simulink model "project"  (R2018b)
settings: Solver=VariableStepAuto  StartTime=0.0  StopTime=10.0  RelTol=1e-3
libraries: commutil2 x4
(part 1 of 2)
settings Model: Creator=Reza  LastModifiedBy=Rahmat

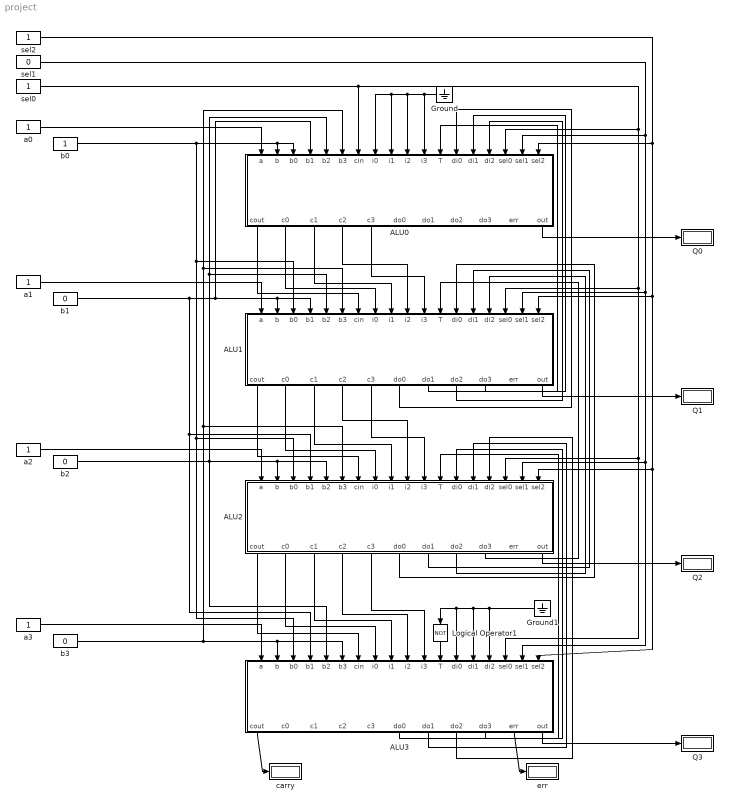
== system project ==
  ALU0 : Subsystem
  ALU1 : Subsystem
  ALU2 : Subsystem
  ALU3 : Subsystem
  Ground : Ground
  Ground1 : Ground
  Logical Operator1 : Logic  Operator=NOT  IconShape=distinctive  AllPortsSameDT=off  OutDataTypeStr=boolean
  Q{0..3} (4 alike) : Display
  a{0..3} (4 alike) : Constant
  b0 : Constant
  b1 : Constant  Value=0
  b2 : Constant  Value=0
  b3 : Constant  Value=0
  carry : Display
  err : Display
  sel0 : Constant
  sel1 : Constant  Value=0
  sel2 : Constant
  wires:
  ALU0/11(out) -> Q0/1
  sel0/1 -> ALU0/7(cin), ALU0/16(sel0), ALU1/16(sel0), ALU2/16(sel0), ALU3/16(sel0)
  sel1/1 -> ALU0/17(sel1), ALU1/17(sel1), ALU2/17(sel1), ALU3/17(sel1)
  sel2/1 -> ALU0/18(sel2), ALU1/18(sel2), ALU2/18(sel2), ALU3/18(sel2)
  ALU1/11(out) -> Q1/1
  ALU2/11(out) -> Q2/1
  ALU3/11(out) -> Q3/1
  a0/1 -> ALU0/1(a)
  a1/1 -> ALU1/1(a)
  a2/1 -> ALU2/1(a)
  a3/1 -> ALU3/1(a)
  b0/1 -> ALU3/3(b0), ALU2/3(b0), ALU1/3(b0), ALU0/3(b0), ALU0/2(b)
  b2/1 -> ALU2/5(b2), ALU2/2(b), ALU3/5(b2), ALU0/5(b2), ALU1/5(b2)
  b3/1 -> ALU3/6(b3), ALU3/2(b), ALU2/6(b3), ALU0/6(b3), ALU1/6(b3)
  b1/1 -> ALU1/4(b1), ALU1/2(b), ALU0/4(b1), ALU3/4(b1), ALU2/4(b1)
  ALU0/1(cout) -> ALU1/7(cin)
  ALU1/1(cout) -> ALU2/7(cin)
  ALU2/1(cout) -> ALU3/7(cin)
  ALU3/1(cout) -> carry/1
  ALU3/10(err) -> err/1
  ALU0/2(c0) -> ALU1/8(i0)
  ALU0/3(c1) -> ALU1/9(i1)
  ALU0/4(c2) -> ALU1/10(i2)
  ALU0/5(c3) -> ALU1/11(i3)
  ALU1/2(c0) -> ALU2/8(i0)
  ALU1/3(c1) -> ALU2/9(i1)
  ALU1/4(c2) -> ALU2/10(i2)
  ALU1/5(c3) -> ALU2/11(i3)
  ALU2/2(c0) -> ALU3/8(i0)
  ALU2/3(c1) -> ALU3/9(i1)
  ALU2/4(c2) -> ALU3/10(i2)
  ALU2/5(c3) -> ALU3/11(i3)
  Ground/1 -> ALU0/11(i3), ALU0/10(i2), ALU0/9(i1), ALU0/8(i0)
  Ground1/1 -> ALU3/14(di1), ALU3/13(di0), Logical Operator1/1, ALU3/15(di2)
  Logical Operator1/1 -> ALU3/12(T)
  ALU3/9(do3) -> ALU2/12(T)
  ALU3/6(do0) -> ALU2/13(di0)
  ALU3/7(do1) -> ALU2/14(di1)
  ALU3/8(do2) -> ALU2/15(di2)
  ALU2/9(do3) -> ALU1/12(T)
  ALU2/8(do2) -> ALU1/15(di2)
  ALU2/7(do1) -> ALU1/14(di1)
  ALU2/6(do0) -> ALU1/13(di0)
  ALU1/9(do3) -> ALU0/12(T)
  ALU1/8(do2) -> ALU0/15(di2)
  ALU1/7(do1) -> ALU0/14(di1)
  ALU1/6(do0) -> ALU0/13(di0)

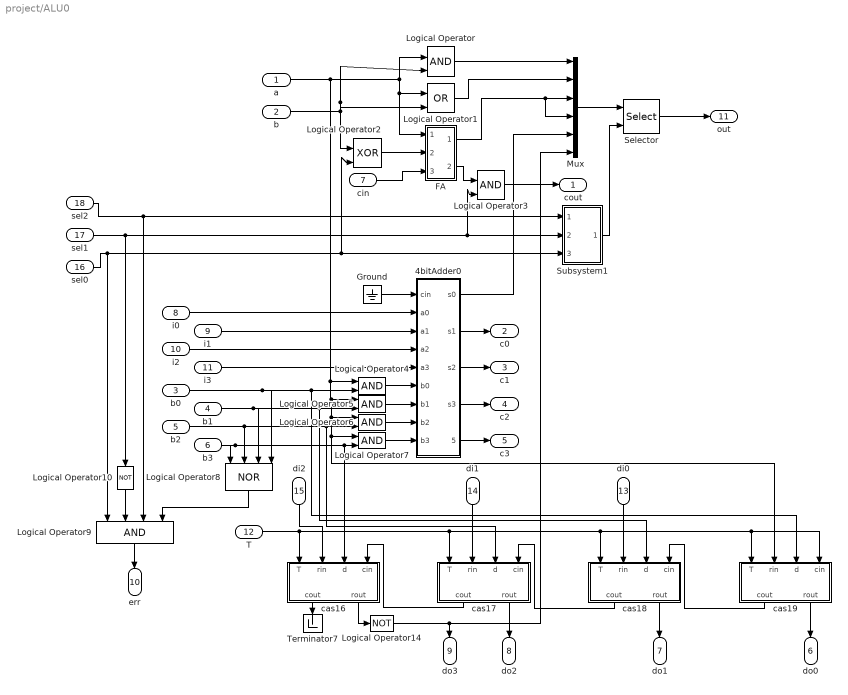
== system project/ALU0 ==
  a : Inport
  b : Inport  Port=2
  b0 : Inport  Port=3
  b1 : Inport  Port=4
  b2 : Inport  Port=5
  b3 : Inport  Port=6
  cin : Inport  Port=7
  i0 : Inport  Port=8
  i1 : Inport  Port=9
  i2 : Inport  Port=10
  i3 : Inport  Port=11
  T : Inport  Port=12
  di0 : Inport  Port=13
  di1 : Inport  Port=14
  di2 : Inport  Port=15
  sel0 : Inport  Port=16
  sel1 : Inport  Port=17
  sel2 : Inport  Port=18
  4bitAdder0 : Subsystem
  FA : Subsystem
  Ground : Ground
  Logical Operator{,3..7} (6 alike) : Logic  IconShape=distinctive  AllPortsSameDT=off  OutDataTypeStr=boolean
  Logical Operator1 : Logic  Operator=OR  IconShape=distinctive  AllPortsSameDT=off  OutDataTypeStr=boolean
  Logical Operator10 : Logic  Operator=NOT  IconShape=distinctive  AllPortsSameDT=off  OutDataTypeStr=boolean
  Logical Operator14 : Logic  Operator=NOT  IconShape=distinctive  AllPortsSameDT=off  OutDataTypeStr=boolean
  Logical Operator2 : Logic  Operator=XOR  IconShape=distinctive  AllPortsSameDT=off  OutDataTypeStr=boolean
  Logical Operator8 : Logic  Operator=NOR  Inputs=4  IconShape=distinctive  AllPortsSameDT=off  OutDataTypeStr=boolean
  Logical Operator9 : Logic  Inputs=4  IconShape=distinctive  AllPortsSameDT=off  OutDataTypeStr=boolean
  Mux : Mux  Inputs=6
  Selector : Selector  InputPortWidth=6  IndexOptions=Starting index (port)  Indices=[1 3]  OutputSizes=1
  Subsystem1 : Subsystem
  Terminator7 : Terminator
  cas16 : Subsystem
  cas17 : Subsystem
  cas18 : Subsystem
  cas19 : Subsystem
  cout : Outport
  c0 : Outport  Port=2
  c1 : Outport  Port=3
  c2 : Outport  Port=4
  c3 : Outport  Port=5
  do0 : Outport  Port=6
  do1 : Outport  Port=7
  do2 : Outport  Port=8
  do3 : Outport  Port=9
  err : Outport  Port=10
  out : Outport  Port=11
  wires:
  b/1 -> Logical Operator/2, Logical Operator1/2, Logical Operator2/1
  Mux/1 -> Selector/1
  sel1/1 -> Logical Operator10/1, Logical Operator3/2, Subsystem1/2(sel1)
  FA/1(Out2) -> Mux/3, Mux/4
  sel2/1 -> Logical Operator9/3, Subsystem1/1(sel2)
  Subsystem1/1(Out1) -> Selector/2
  a/1 -> Logical Operator7/1, cas19/2(rin), Logical Operator6/1, Logical Operator5/1, Logical Operator4/1, FA/1(In2), Logical Operator1/1, Logical Operator/1
  cin/1 -> FA/3(In4)
  Logical Operator2/1 -> FA/2(In3)
  Selector/1 -> out/1
  sel0/1 -> Logical Operator9/1, Logical Operator2/2, Subsystem1/3(sel0)
  Logical Operator1/1 -> Mux/2
  Logical Operator/1 -> Mux/1
  FA/2(Out1) -> Logical Operator3/1
  Logical Operator3/1 -> cout/1
  4bitAdder0/1(s0) -> Mux/5
  i0/1 -> 4bitAdder0/2(a0)
  i1/1 -> 4bitAdder0/3(a1)
  i2/1 -> 4bitAdder0/4(a2)
  i3/1 -> 4bitAdder0/5(a3)
  Logical Operator4/1 -> 4bitAdder0/6(b0)
  Logical Operator5/1 -> 4bitAdder0/7(b1)
  4bitAdder0/2(s1) -> c0/1
  4bitAdder0/3(s2) -> c1/1
  4bitAdder0/4(s3) -> c2/1
  4bitAdder0/5(cout) -> c3/1
  Logical Operator6/1 -> 4bitAdder0/8(b2)
  Logical Operator7/1 -> 4bitAdder0/9(b3)
  b0/1 -> Logical Operator8/4, Logical Operator4/2, cas19/3(d)
  b1/1 -> Logical Operator8/3, Logical Operator5/2, cas18/3(d)
  b2/1 -> Logical Operator8/2, cas17/3(d), Logical Operator6/2
  b3/1 -> Logical Operator8/1, cas16/3(d), Logical Operator7/2
  cas19/1(cout) -> cas18/4(cin)
  cas18/1(cout) -> cas17/4(cin)
  cas17/1(cout) -> cas16/4(cin)
  cas16/1(cout) -> Terminator7/1
  T/1 -> cas16/1(T), cas17/1(T), cas18/1(T), cas19/1(T), cas19/4(cin)
  cas16/2(rout) -> Logical Operator14/1
  Logical Operator14/1 -> do3/1, Mux/6
  di0/1 -> cas18/2(rin)
  di1/1 -> cas17/2(rin)
  di2/1 -> cas16/2(rin)
  cas19/2(rout) -> do0/1
  cas18/2(rout) -> do1/1
  cas17/2(rout) -> do2/1
  Ground/1 -> 4bitAdder0/1(cin)
  Logical Operator9/1 -> err/1
  Logical Operator8/1 -> Logical Operator9/4
  Logical Operator10/1 -> Logical Operator9/2

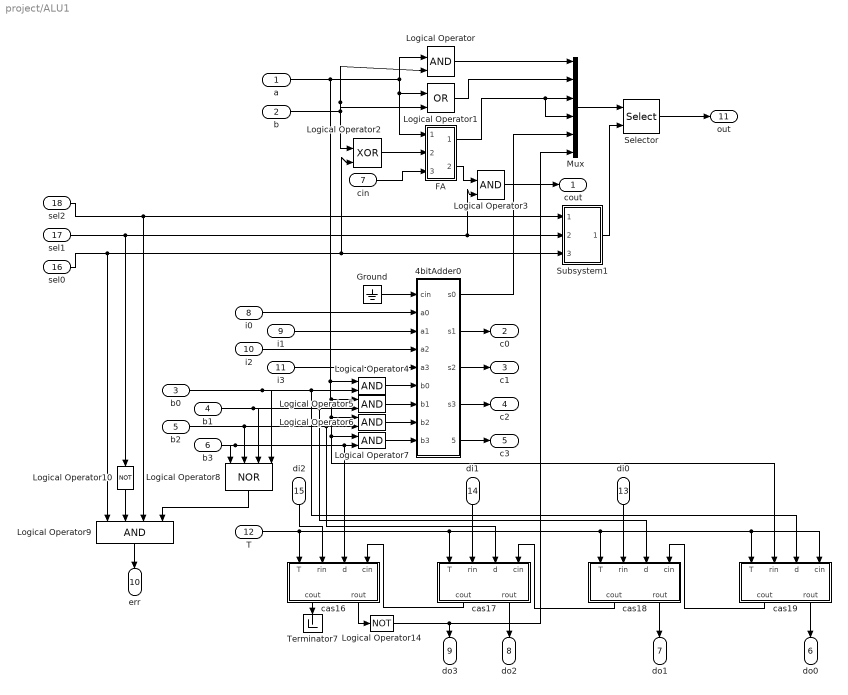
== system project/ALU1 ==
  a : Inport
  b : Inport  Port=2
  b0 : Inport  Port=3
  b1 : Inport  Port=4
  b2 : Inport  Port=5
  b3 : Inport  Port=6
  cin : Inport  Port=7
  i0 : Inport  Port=8
  i1 : Inport  Port=9
  i2 : Inport  Port=10
  i3 : Inport  Port=11
  T : Inport  Port=12
  di0 : Inport  Port=13
  di1 : Inport  Port=14
  di2 : Inport  Port=15
  sel0 : Inport  Port=16
  sel1 : Inport  Port=17
  sel2 : Inport  Port=18
  4bitAdder0 : Subsystem
  FA : Subsystem
  Ground : Ground
  Logical Operator{,3..7} (6 alike) : Logic  IconShape=distinctive  AllPortsSameDT=off  OutDataTypeStr=boolean
  Logical Operator1 : Logic  Operator=OR  IconShape=distinctive  AllPortsSameDT=off  OutDataTypeStr=boolean
  Logical Operator10 : Logic  Operator=NOT  IconShape=distinctive  AllPortsSameDT=off  OutDataTypeStr=boolean
  Logical Operator14 : Logic  Operator=NOT  IconShape=distinctive  AllPortsSameDT=off  OutDataTypeStr=boolean
  Logical Operator2 : Logic  Operator=XOR  IconShape=distinctive  AllPortsSameDT=off  OutDataTypeStr=boolean
  Logical Operator8 : Logic  Operator=NOR  Inputs=4  IconShape=distinctive  AllPortsSameDT=off  OutDataTypeStr=boolean
  Logical Operator9 : Logic  Inputs=4  IconShape=distinctive  AllPortsSameDT=off  OutDataTypeStr=boolean
  Mux : Mux  Inputs=6
  Selector : Selector  InputPortWidth=6  IndexOptions=Starting index (port)  Indices=[1 3]  OutputSizes=1
  Subsystem1 : Subsystem
  Terminator7 : Terminator
  cas16 : Subsystem
  cas17 : Subsystem
  cas18 : Subsystem
  cas19 : Subsystem
  cout : Outport
  c0 : Outport  Port=2
  c1 : Outport  Port=3
  c2 : Outport  Port=4
  c3 : Outport  Port=5
  do0 : Outport  Port=6
  do1 : Outport  Port=7
  do2 : Outport  Port=8
  do3 : Outport  Port=9
  err : Outport  Port=10
  out : Outport  Port=11
  wires:
  b/1 -> Logical Operator/2, Logical Operator1/2, Logical Operator2/1
  Mux/1 -> Selector/1
  FA/1(Out2) -> Mux/3, Mux/4
  Subsystem1/1(Out1) -> Selector/2
  a/1 -> Logical Operator7/1, cas19/2(rin), Logical Operator6/1, Logical Operator5/1, Logical Operator4/1, FA/1(In2), Logical Operator1/1, Logical Operator/1
  cin/1 -> FA/3(In4)
  Logical Operator2/1 -> FA/2(In3)
  Selector/1 -> out/1
  Logical Operator1/1 -> Mux/2
  Logical Operator/1 -> Mux/1
  FA/2(Out1) -> Logical Operator3/1
  Logical Operator3/1 -> cout/1
  4bitAdder0/1(s0) -> Mux/5
  i0/1 -> 4bitAdder0/2(a0)
  i1/1 -> 4bitAdder0/3(a1)
  i2/1 -> 4bitAdder0/4(a2)
  i3/1 -> 4bitAdder0/5(a3)
  Logical Operator4/1 -> 4bitAdder0/6(b0)
  Logical Operator5/1 -> 4bitAdder0/7(b1)
  4bitAdder0/2(s1) -> c0/1
  4bitAdder0/3(s2) -> c1/1
  4bitAdder0/4(s3) -> c2/1
  4bitAdder0/5(cout) -> c3/1
  Logical Operator6/1 -> 4bitAdder0/8(b2)
  Logical Operator7/1 -> 4bitAdder0/9(b3)
  b0/1 -> Logical Operator8/4, Logical Operator4/2, cas19/3(d)
  b1/1 -> Logical Operator8/3, Logical Operator5/2, cas18/3(d)
  b2/1 -> Logical Operator8/2, cas17/3(d), Logical Operator6/2
  b3/1 -> Logical Operator8/1, cas16/3(d), Logical Operator7/2
  cas19/1(cout) -> cas18/4(cin)
  cas18/1(cout) -> cas17/4(cin)
  cas17/1(cout) -> cas16/4(cin)
  cas16/1(cout) -> Terminator7/1
  T/1 -> cas16/1(T), cas17/1(T), cas18/1(T), cas19/1(T), cas19/4(cin)
  cas16/2(rout) -> Logical Operator14/1
  Logical Operator14/1 -> do3/1, Mux/6
  di0/1 -> cas18/2(rin)
  di1/1 -> cas17/2(rin)
  di2/1 -> cas16/2(rin)
  cas19/2(rout) -> do0/1
  cas18/2(rout) -> do1/1
  cas17/2(rout) -> do2/1
  Ground/1 -> 4bitAdder0/1(cin)
  sel2/1 -> Logical Operator9/3, Subsystem1/1(sel2)
  sel0/1 -> Logical Operator9/1, Logical Operator2/2, Subsystem1/3(sel0)
  Logical Operator10/1 -> Logical Operator9/2
  Logical Operator9/1 -> err/1
  Logical Operator8/1 -> Logical Operator9/4
  sel1/1 -> Logical Operator10/1, Logical Operator3/2, Subsystem1/2(sel1)

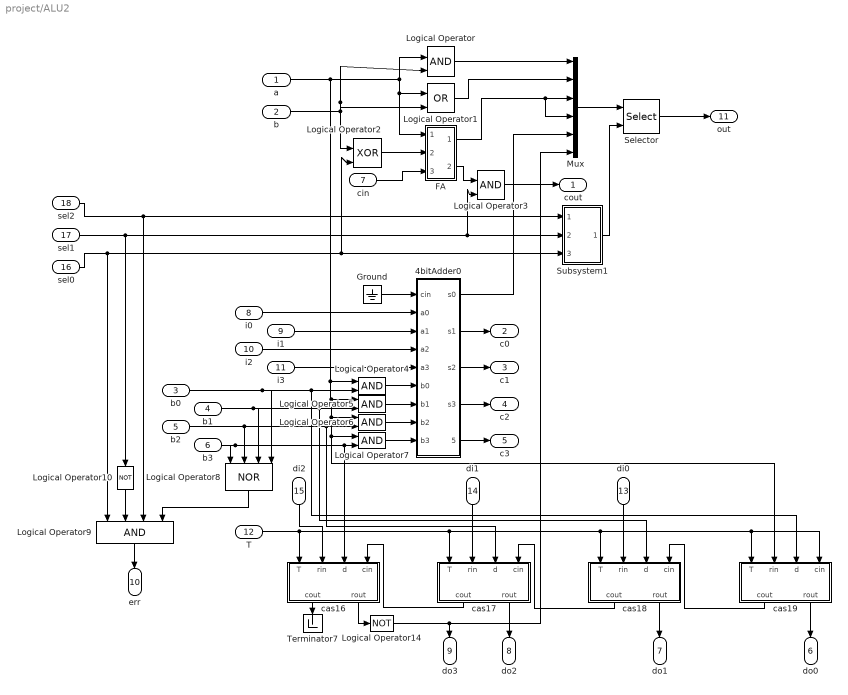
== system project/ALU2 ==
  a : Inport
  b : Inport  Port=2
  b0 : Inport  Port=3
  b1 : Inport  Port=4
  b2 : Inport  Port=5
  b3 : Inport  Port=6
  cin : Inport  Port=7
  i0 : Inport  Port=8
  i1 : Inport  Port=9
  i2 : Inport  Port=10
  i3 : Inport  Port=11
  T : Inport  Port=12
  di0 : Inport  Port=13
  di1 : Inport  Port=14
  di2 : Inport  Port=15
  sel0 : Inport  Port=16
  sel1 : Inport  Port=17
  sel2 : Inport  Port=18
  4bitAdder0 : Subsystem
  FA : Subsystem
  Ground : Ground
  Logical Operator{,3..7} (6 alike) : Logic  IconShape=distinctive  AllPortsSameDT=off  OutDataTypeStr=boolean
  Logical Operator1 : Logic  Operator=OR  IconShape=distinctive  AllPortsSameDT=off  OutDataTypeStr=boolean
  Logical Operator10 : Logic  Operator=NOT  IconShape=distinctive  AllPortsSameDT=off  OutDataTypeStr=boolean
  Logical Operator14 : Logic  Operator=NOT  IconShape=distinctive  AllPortsSameDT=off  OutDataTypeStr=boolean
  Logical Operator2 : Logic  Operator=XOR  IconShape=distinctive  AllPortsSameDT=off  OutDataTypeStr=boolean
  Logical Operator8 : Logic  Operator=NOR  Inputs=4  IconShape=distinctive  AllPortsSameDT=off  OutDataTypeStr=boolean
  Logical Operator9 : Logic  Inputs=4  IconShape=distinctive  AllPortsSameDT=off  OutDataTypeStr=boolean
  Mux : Mux  Inputs=6
  Selector : Selector  InputPortWidth=6  IndexOptions=Starting index (port)  Indices=[1 3]  OutputSizes=1
  Subsystem1 : Subsystem
  Terminator7 : Terminator
  cas16 : Subsystem
  cas17 : Subsystem
  cas18 : Subsystem
  cas19 : Subsystem
  cout : Outport
  c0 : Outport  Port=2
  c1 : Outport  Port=3
  c2 : Outport  Port=4
  c3 : Outport  Port=5
  do0 : Outport  Port=6
  do1 : Outport  Port=7
  do2 : Outport  Port=8
  do3 : Outport  Port=9
  err : Outport  Port=10
  out : Outport  Port=11
  wires:
  b/1 -> Logical Operator/2, Logical Operator1/2, Logical Operator2/1
  Mux/1 -> Selector/1
  FA/1(Out2) -> Mux/3, Mux/4
  Subsystem1/1(Out1) -> Selector/2
  a/1 -> Logical Operator7/1, cas19/2(rin), Logical Operator6/1, Logical Operator5/1, Logical Operator4/1, FA/1(In2), Logical Operator1/1, Logical Operator/1
  cin/1 -> FA/3(In4)
  Logical Operator2/1 -> FA/2(In3)
  Selector/1 -> out/1
  Logical Operator1/1 -> Mux/2
  Logical Operator/1 -> Mux/1
  FA/2(Out1) -> Logical Operator3/1
  Logical Operator3/1 -> cout/1
  4bitAdder0/1(s0) -> Mux/5
  i0/1 -> 4bitAdder0/2(a0)
  i1/1 -> 4bitAdder0/3(a1)
  i2/1 -> 4bitAdder0/4(a2)
  i3/1 -> 4bitAdder0/5(a3)
  Logical Operator4/1 -> 4bitAdder0/6(b0)
  Logical Operator5/1 -> 4bitAdder0/7(b1)
  4bitAdder0/2(s1) -> c0/1
  4bitAdder0/3(s2) -> c1/1
  4bitAdder0/4(s3) -> c2/1
  4bitAdder0/5(cout) -> c3/1
  Logical Operator6/1 -> 4bitAdder0/8(b2)
  Logical Operator7/1 -> 4bitAdder0/9(b3)
  b0/1 -> Logical Operator8/4, Logical Operator4/2, cas19/3(d)
  b1/1 -> Logical Operator8/3, Logical Operator5/2, cas18/3(d)
  b2/1 -> Logical Operator8/2, cas17/3(d), Logical Operator6/2
  b3/1 -> Logical Operator8/1, cas16/3(d), Logical Operator7/2
  cas19/1(cout) -> cas18/4(cin)
  cas18/1(cout) -> cas17/4(cin)
  cas17/1(cout) -> cas16/4(cin)
  cas16/1(cout) -> Terminator7/1
  T/1 -> cas16/1(T), cas17/1(T), cas18/1(T), cas19/1(T), cas19/4(cin)
  cas16/2(rout) -> Logical Operator14/1
  Logical Operator14/1 -> do3/1, Mux/6
  di0/1 -> cas18/2(rin)
  di1/1 -> cas17/2(rin)
  di2/1 -> cas16/2(rin)
  cas19/2(rout) -> do0/1
  cas18/2(rout) -> do1/1
  cas17/2(rout) -> do2/1
  Ground/1 -> 4bitAdder0/1(cin)
  sel2/1 -> Subsystem1/1(sel2), Logical Operator9/3
  sel0/1 -> Logical Operator9/1, Logical Operator2/2, Subsystem1/3(sel0)
  Logical Operator10/1 -> Logical Operator9/2
  Logical Operator9/1 -> err/1
  Logical Operator8/1 -> Logical Operator9/4
  sel1/1 -> Logical Operator3/2, Subsystem1/2(sel1), Logical Operator10/1

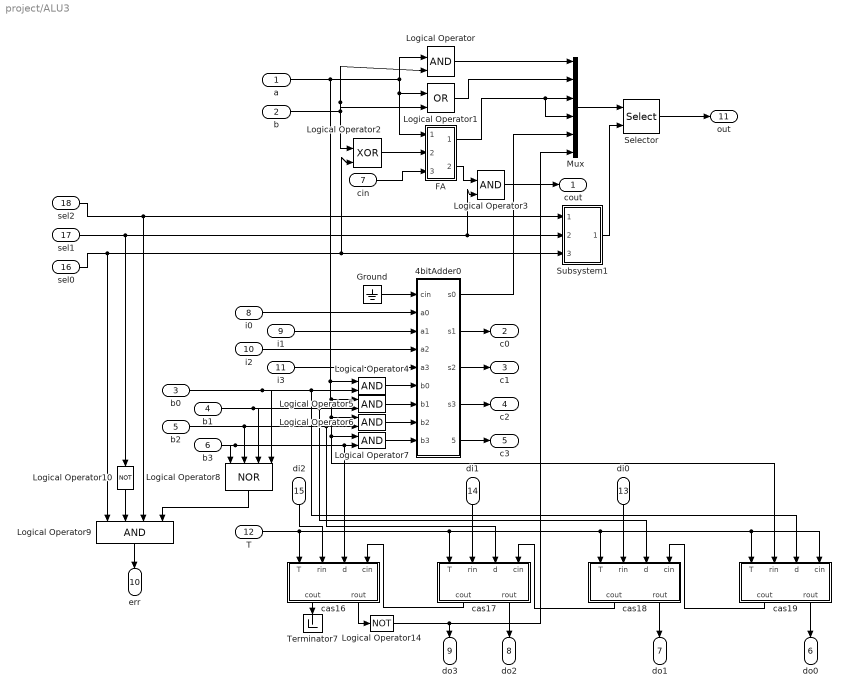
== system project/ALU3 ==
  a : Inport
  b : Inport  Port=2
  b0 : Inport  Port=3
  b1 : Inport  Port=4
  b2 : Inport  Port=5
  b3 : Inport  Port=6
  cin : Inport  Port=7
  i0 : Inport  Port=8
  i1 : Inport  Port=9
  i2 : Inport  Port=10
  i3 : Inport  Port=11
  T : Inport  Port=12
  di0 : Inport  Port=13
  di1 : Inport  Port=14
  di2 : Inport  Port=15
  sel0 : Inport  Port=16
  sel1 : Inport  Port=17
  sel2 : Inport  Port=18
  4bitAdder0 : Subsystem
  FA : Subsystem
  Ground : Ground
  Logical Operator{,3..7} (6 alike) : Logic  IconShape=distinctive  AllPortsSameDT=off  OutDataTypeStr=boolean
  Logical Operator1 : Logic  Operator=OR  IconShape=distinctive  AllPortsSameDT=off  OutDataTypeStr=boolean
  Logical Operator10 : Logic  Operator=NOT  IconShape=distinctive  AllPortsSameDT=off  OutDataTypeStr=boolean
  Logical Operator14 : Logic  Operator=NOT  IconShape=distinctive  AllPortsSameDT=off  OutDataTypeStr=boolean
  Logical Operator2 : Logic  Operator=XOR  IconShape=distinctive  AllPortsSameDT=off  OutDataTypeStr=boolean
  Logical Operator8 : Logic  Operator=NOR  Inputs=4  IconShape=distinctive  AllPortsSameDT=off  OutDataTypeStr=boolean
  Logical Operator9 : Logic  Inputs=4  IconShape=distinctive  AllPortsSameDT=off  OutDataTypeStr=boolean
  Mux : Mux  Inputs=6
  Selector : Selector  InputPortWidth=6  IndexOptions=Starting index (port)  Indices=[1 3]  OutputSizes=1
  Subsystem1 : Subsystem
  Terminator7 : Terminator
  cas16 : Subsystem
  cas17 : Subsystem
  cas18 : Subsystem
  cas19 : Subsystem
  cout : Outport
  c0 : Outport  Port=2
  c1 : Outport  Port=3
  c2 : Outport  Port=4
  c3 : Outport  Port=5
  do0 : Outport  Port=6
  do1 : Outport  Port=7
  do2 : Outport  Port=8
  do3 : Outport  Port=9
  err : Outport  Port=10
  out : Outport  Port=11
  wires:
  b/1 -> Logical Operator/2, Logical Operator1/2, Logical Operator2/1
  Mux/1 -> Selector/1
  FA/1(Out2) -> Mux/3, Mux/4
  Subsystem1/1(Out1) -> Selector/2
  a/1 -> Logical Operator7/1, cas19/2(rin), Logical Operator6/1, Logical Operator5/1, Logical Operator4/1, FA/1(In2), Logical Operator1/1, Logical Operator/1
  cin/1 -> FA/3(In4)
  Logical Operator2/1 -> FA/2(In3)
  Selector/1 -> out/1
  Logical Operator1/1 -> Mux/2
  Logical Operator/1 -> Mux/1
  FA/2(Out1) -> Logical Operator3/1
  Logical Operator3/1 -> cout/1
  4bitAdder0/1(s0) -> Mux/5
  i0/1 -> 4bitAdder0/2(a0)
  i1/1 -> 4bitAdder0/3(a1)
  i2/1 -> 4bitAdder0/4(a2)
  i3/1 -> 4bitAdder0/5(a3)
  Logical Operator4/1 -> 4bitAdder0/6(b0)
  Logical Operator5/1 -> 4bitAdder0/7(b1)
  4bitAdder0/2(s1) -> c0/1
  4bitAdder0/3(s2) -> c1/1
  4bitAdder0/4(s3) -> c2/1
  4bitAdder0/5(cout) -> c3/1
  Logical Operator6/1 -> 4bitAdder0/8(b2)
  Logical Operator7/1 -> 4bitAdder0/9(b3)
  b0/1 -> Logical Operator8/4, Logical Operator4/2, cas19/3(d)
  b1/1 -> Logical Operator8/3, Logical Operator5/2, cas18/3(d)
  b2/1 -> Logical Operator8/2, cas17/3(d), Logical Operator6/2
  b3/1 -> Logical Operator8/1, cas16/3(d), Logical Operator7/2
  cas19/1(cout) -> cas18/4(cin)
  cas18/1(cout) -> cas17/4(cin)
  cas17/1(cout) -> cas16/4(cin)
  cas16/1(cout) -> Terminator7/1
  T/1 -> cas16/1(T), cas17/1(T), cas18/1(T), cas19/1(T), cas19/4(cin)
  cas16/2(rout) -> Logical Operator14/1
  Logical Operator14/1 -> do3/1, Mux/6
  di0/1 -> cas18/2(rin)
  di1/1 -> cas17/2(rin)
  di2/1 -> cas16/2(rin)
  cas19/2(rout) -> do0/1
  cas18/2(rout) -> do1/1
  cas17/2(rout) -> do2/1
  Ground/1 -> 4bitAdder0/1(cin)
  sel2/1 -> Logical Operator9/3, Subsystem1/1(sel2)
  sel0/1 -> Logical Operator9/1, Logical Operator2/2, Subsystem1/3(sel0)
  Logical Operator10/1 -> Logical Operator9/2
  Logical Operator9/1 -> err/1
  Logical Operator8/1 -> Logical Operator9/4
  sel1/1 -> Logical Operator10/1, Logical Operator3/2, Subsystem1/2(sel1)

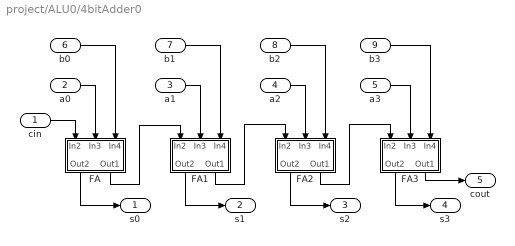
== system project/ALU0/4bitAdder0 ==
  cin : Inport
  a0 : Inport  Port=2
  a1 : Inport  Port=3
  a2 : Inport  Port=4
  a3 : Inport  Port=5
  b0 : Inport  Port=6
  b1 : Inport  Port=7
  b2 : Inport  Port=8
  b3 : Inport  Port=9
  FA : Subsystem
  FA1 : Subsystem
  FA2 : Subsystem
  FA3 : Subsystem
  s0 : Outport
  s1 : Outport  Port=2
  s2 : Outport  Port=3
  s3 : Outport  Port=4
  cout : Outport  Port=5
  wires:
  a2/1 -> FA2/2(In3)
  a0/1 -> FA/2(In3)
  FA2/2(Out1) -> FA3/1(In2)
  b2/1 -> FA2/3(In4)
  b3/1 -> FA3/3(In4)
  cin/1 -> FA/1(In2)
  a3/1 -> FA3/2(In3)
  FA2/1(Out2) -> s2/1
  FA3/1(Out2) -> s3/1
  FA/1(Out2) -> s0/1
  b0/1 -> FA/3(In4)
  a1/1 -> FA1/2(In3)
  FA1/1(Out2) -> s1/1
  FA/2(Out1) -> FA1/1(In2)
  b1/1 -> FA1/3(In4)
  FA1/2(Out1) -> FA2/1(In2)
  FA3/2(Out1) -> cout/1

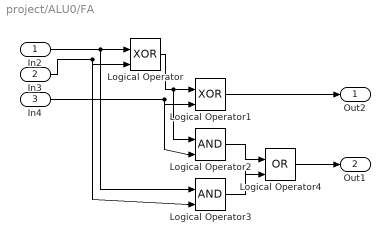
== system project/ALU0/FA ==
  In2 : Inport
  In3 : Inport  Port=2
  In4 : Inport  Port=3
  Logical Operator : Logic  Operator=XOR  IconShape=distinctive  AllPortsSameDT=off  OutDataTypeStr=boolean
  Logical Operator1 : Logic  Operator=XOR  IconShape=distinctive  AllPortsSameDT=off  OutDataTypeStr=boolean
  Logical Operator2 : Logic  IconShape=distinctive  AllPortsSameDT=off  OutDataTypeStr=boolean
  Logical Operator3 : Logic  IconShape=distinctive  AllPortsSameDT=off  OutDataTypeStr=boolean
  Logical Operator4 : Logic  Operator=OR  IconShape=distinctive  AllPortsSameDT=off  OutDataTypeStr=boolean
  Out2 : Outport
  Out1 : Outport  Port=2
  wires:
  In2/1 -> Logical Operator3/1, Logical Operator/1
  In3/1 -> Logical Operator3/2, Logical Operator/2
  Logical Operator/1 -> Logical Operator1/1, Logical Operator2/1
  Logical Operator1/1 -> Out2/1
  Logical Operator4/1 -> Out1/1
  Logical Operator2/1 -> Logical Operator4/1
  Logical Operator3/1 -> Logical Operator4/2
  In4/1 -> Logical Operator2/2, Logical Operator1/2

== system project/ALU0/Subsystem1 ==
  sel2 : Inport
  sel1 : Inport  Port=2
  sel0 : Inport  Port=3
  Add : Sum
  Bit to Integer Converter : commutil2/Bit to Integer Converter  nbits=3  bitOrder=MSB first  signedOutputValues=Unsigned  outDtype=Inherit via internal rule  outDtypeSigned=Inherit via internal rule
  Ground : Ground
  Logical Operator3 : Logic  Operator=NOT  IconShape=distinctive  AllPortsSameDT=off  OutDataTypeStr=boolean
  Mux1 : Mux  Inputs=3
  Out1 : Outport
  wires:
  sel0/1 -> Mux1/3
  Ground/1 -> Logical Operator3/1
  Bit to Integer Converter/1 -> Add/1
  sel1/1 -> Mux1/2
  Mux1/1 -> Bit to Integer Converter/1
  Add/1 -> Out1/1
  Logical Operator3/1 -> Add/2
  sel2/1 -> Mux1/1

== system project/ALU0/cas16 ==
  T : Inport
  rin : Inport  Port=2
  d : Inport  Port=3
  cin : Inport  Port=4
  FA : Subsystem
  Logical Operator : Logic  Operator=XOR  IconShape=distinctive  AllPortsSameDT=off  OutDataTypeStr=boolean
  cout : Outport
  rout : Outport  Port=2
  wires:
  cin/1 -> FA/3(In4)
  rin/1 -> FA/1(In2)
  FA/2(Out1) -> cout/1
  T/1 -> Logical Operator/1
  d/1 -> Logical Operator/2
  Logical Operator/1 -> FA/2(In3)
  FA/1(Out2) -> rout/1

== system project/ALU0/cas17 ==
  T : Inport
  rin : Inport  Port=2
  d : Inport  Port=3
  cin : Inport  Port=4
  FA : Subsystem
  Logical Operator : Logic  Operator=XOR  IconShape=distinctive  AllPortsSameDT=off  OutDataTypeStr=boolean
  cout : Outport
  rout : Outport  Port=2
  wires:
  cin/1 -> FA/3(In4)
  rin/1 -> FA/1(In2)
  FA/2(Out1) -> cout/1
  T/1 -> Logical Operator/1
  d/1 -> Logical Operator/2
  Logical Operator/1 -> FA/2(In3)
  FA/1(Out2) -> rout/1

== system project/ALU0/cas18 ==
  T : Inport
  rin : Inport  Port=2
  d : Inport  Port=3
  cin : Inport  Port=4
  FA : Subsystem
  Logical Operator : Logic  Operator=XOR  IconShape=distinctive  AllPortsSameDT=off  OutDataTypeStr=boolean
  cout : Outport
  rout : Outport  Port=2
  wires:
  cin/1 -> FA/3(In4)
  rin/1 -> FA/1(In2)
  FA/2(Out1) -> cout/1
  T/1 -> Logical Operator/1
  d/1 -> Logical Operator/2
  Logical Operator/1 -> FA/2(In3)
  FA/1(Out2) -> rout/1

== system project/ALU0/cas19 ==
  T : Inport
  rin : Inport  Port=2
  d : Inport  Port=3
  cin : Inport  Port=4
  FA : Subsystem
  Logical Operator : Logic  Operator=XOR  IconShape=distinctive  AllPortsSameDT=off  OutDataTypeStr=boolean
  cout : Outport
  rout : Outport  Port=2
  wires:
  cin/1 -> FA/3(In4)
  rin/1 -> FA/1(In2)
  FA/2(Out1) -> cout/1
  T/1 -> Logical Operator/1
  d/1 -> Logical Operator/2
  Logical Operator/1 -> FA/2(In3)
  FA/1(Out2) -> rout/1

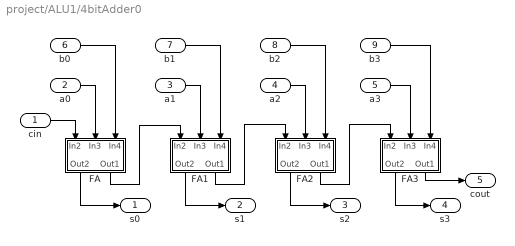
== system project/ALU1/4bitAdder0 ==
  cin : Inport
  a0 : Inport  Port=2
  a1 : Inport  Port=3
  a2 : Inport  Port=4
  a3 : Inport  Port=5
  b0 : Inport  Port=6
  b1 : Inport  Port=7
  b2 : Inport  Port=8
  b3 : Inport  Port=9
  FA : Subsystem
  FA1 : Subsystem
  FA2 : Subsystem
  FA3 : Subsystem
  s0 : Outport
  s1 : Outport  Port=2
  s2 : Outport  Port=3
  s3 : Outport  Port=4
  cout : Outport  Port=5
  wires:
  a2/1 -> FA2/2(In3)
  a0/1 -> FA/2(In3)
  FA2/2(Out1) -> FA3/1(In2)
  b2/1 -> FA2/3(In4)
  b3/1 -> FA3/3(In4)
  cin/1 -> FA/1(In2)
  a3/1 -> FA3/2(In3)
  FA2/1(Out2) -> s2/1
  FA3/1(Out2) -> s3/1
  FA/1(Out2) -> s0/1
  b0/1 -> FA/3(In4)
  a1/1 -> FA1/2(In3)
  FA1/1(Out2) -> s1/1
  FA/2(Out1) -> FA1/1(In2)
  b1/1 -> FA1/3(In4)
  FA1/2(Out1) -> FA2/1(In2)
  FA3/2(Out1) -> cout/1

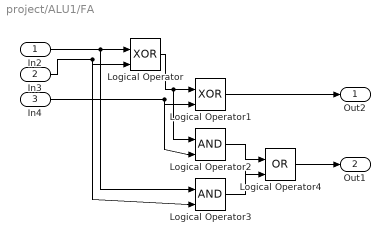
== system project/ALU1/FA ==
  In2 : Inport
  In3 : Inport  Port=2
  In4 : Inport  Port=3
  Logical Operator : Logic  Operator=XOR  IconShape=distinctive  AllPortsSameDT=off  OutDataTypeStr=boolean
  Logical Operator1 : Logic  Operator=XOR  IconShape=distinctive  AllPortsSameDT=off  OutDataTypeStr=boolean
  Logical Operator2 : Logic  IconShape=distinctive  AllPortsSameDT=off  OutDataTypeStr=boolean
  Logical Operator3 : Logic  IconShape=distinctive  AllPortsSameDT=off  OutDataTypeStr=boolean
  Logical Operator4 : Logic  Operator=OR  IconShape=distinctive  AllPortsSameDT=off  OutDataTypeStr=boolean
  Out2 : Outport
  Out1 : Outport  Port=2
  wires:
  In2/1 -> Logical Operator3/1, Logical Operator/1
  In3/1 -> Logical Operator3/2, Logical Operator/2
  Logical Operator/1 -> Logical Operator1/1, Logical Operator2/1
  Logical Operator1/1 -> Out2/1
  Logical Operator4/1 -> Out1/1
  Logical Operator2/1 -> Logical Operator4/1
  Logical Operator3/1 -> Logical Operator4/2
  In4/1 -> Logical Operator2/2, Logical Operator1/2

== system project/ALU1/Subsystem1 ==
  sel2 : Inport
  sel1 : Inport  Port=2
  sel0 : Inport  Port=3
  Add : Sum
  Bit to Integer Converter : commutil2/Bit to Integer Converter  nbits=3  bitOrder=MSB first  signedOutputValues=Unsigned  outDtype=Inherit via internal rule  outDtypeSigned=Inherit via internal rule
  Ground : Ground
  Logical Operator3 : Logic  Operator=NOT  IconShape=distinctive  AllPortsSameDT=off  OutDataTypeStr=boolean
  Mux1 : Mux  Inputs=3
  Out1 : Outport
  wires:
  sel0/1 -> Mux1/3
  Ground/1 -> Logical Operator3/1
  Bit to Integer Converter/1 -> Add/1
  sel1/1 -> Mux1/2
  Mux1/1 -> Bit to Integer Converter/1
  Add/1 -> Out1/1
  Logical Operator3/1 -> Add/2
  sel2/1 -> Mux1/1

== system project/ALU1/cas16 ==
  T : Inport
  rin : Inport  Port=2
  d : Inport  Port=3
  cin : Inport  Port=4
  FA : Subsystem
  Logical Operator : Logic  Operator=XOR  IconShape=distinctive  AllPortsSameDT=off  OutDataTypeStr=boolean
  cout : Outport
  rout : Outport  Port=2
  wires:
  cin/1 -> FA/3(In4)
  rin/1 -> FA/1(In2)
  FA/2(Out1) -> cout/1
  T/1 -> Logical Operator/1
  d/1 -> Logical Operator/2
  Logical Operator/1 -> FA/2(In3)
  FA/1(Out2) -> rout/1

== system project/ALU1/cas17 ==
  T : Inport
  rin : Inport  Port=2
  d : Inport  Port=3
  cin : Inport  Port=4
  FA : Subsystem
  Logical Operator : Logic  Operator=XOR  IconShape=distinctive  AllPortsSameDT=off  OutDataTypeStr=boolean
  cout : Outport
  rout : Outport  Port=2
  wires:
  cin/1 -> FA/3(In4)
  rin/1 -> FA/1(In2)
  FA/2(Out1) -> cout/1
  T/1 -> Logical Operator/1
  d/1 -> Logical Operator/2
  Logical Operator/1 -> FA/2(In3)
  FA/1(Out2) -> rout/1

== system project/ALU1/cas18 ==
  T : Inport
  rin : Inport  Port=2
  d : Inport  Port=3
  cin : Inport  Port=4
  FA : Subsystem
  Logical Operator : Logic  Operator=XOR  IconShape=distinctive  AllPortsSameDT=off  OutDataTypeStr=boolean
  cout : Outport
  rout : Outport  Port=2
  wires:
  cin/1 -> FA/3(In4)
  rin/1 -> FA/1(In2)
  FA/2(Out1) -> cout/1
  T/1 -> Logical Operator/1
  d/1 -> Logical Operator/2
  Logical Operator/1 -> FA/2(In3)
  FA/1(Out2) -> rout/1

== system project/ALU1/cas19 ==
  T : Inport
  rin : Inport  Port=2
  d : Inport  Port=3
  cin : Inport  Port=4
  FA : Subsystem
  Logical Operator : Logic  Operator=XOR  IconShape=distinctive  AllPortsSameDT=off  OutDataTypeStr=boolean
  cout : Outport
  rout : Outport  Port=2
  wires:
  cin/1 -> FA/3(In4)
  rin/1 -> FA/1(In2)
  FA/2(Out1) -> cout/1
  T/1 -> Logical Operator/1
  d/1 -> Logical Operator/2
  Logical Operator/1 -> FA/2(In3)
  FA/1(Out2) -> rout/1

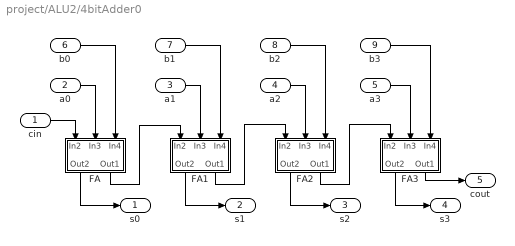
== system project/ALU2/4bitAdder0 ==
  cin : Inport
  a0 : Inport  Port=2
  a1 : Inport  Port=3
  a2 : Inport  Port=4
  a3 : Inport  Port=5
  b0 : Inport  Port=6
  b1 : Inport  Port=7
  b2 : Inport  Port=8
  b3 : Inport  Port=9
  FA : Subsystem
  FA1 : Subsystem
  FA2 : Subsystem
  FA3 : Subsystem
  s0 : Outport
  s1 : Outport  Port=2
  s2 : Outport  Port=3
  s3 : Outport  Port=4
  cout : Outport  Port=5
  wires:
  a2/1 -> FA2/2(In3)
  a0/1 -> FA/2(In3)
  FA2/2(Out1) -> FA3/1(In2)
  b2/1 -> FA2/3(In4)
  b3/1 -> FA3/3(In4)
  cin/1 -> FA/1(In2)
  a3/1 -> FA3/2(In3)
  FA2/1(Out2) -> s2/1
  FA3/1(Out2) -> s3/1
  FA/1(Out2) -> s0/1
  b0/1 -> FA/3(In4)
  a1/1 -> FA1/2(In3)
  FA1/1(Out2) -> s1/1
  FA/2(Out1) -> FA1/1(In2)
  b1/1 -> FA1/3(In4)
  FA1/2(Out1) -> FA2/1(In2)
  FA3/2(Out1) -> cout/1

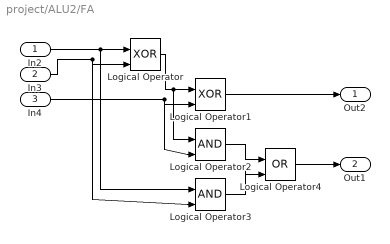
== system project/ALU2/FA ==
  In2 : Inport
  In3 : Inport  Port=2
  In4 : Inport  Port=3
  Logical Operator : Logic  Operator=XOR  IconShape=distinctive  AllPortsSameDT=off  OutDataTypeStr=boolean
  Logical Operator1 : Logic  Operator=XOR  IconShape=distinctive  AllPortsSameDT=off  OutDataTypeStr=boolean
  Logical Operator2 : Logic  IconShape=distinctive  AllPortsSameDT=off  OutDataTypeStr=boolean
  Logical Operator3 : Logic  IconShape=distinctive  AllPortsSameDT=off  OutDataTypeStr=boolean
  Logical Operator4 : Logic  Operator=OR  IconShape=distinctive  AllPortsSameDT=off  OutDataTypeStr=boolean
  Out2 : Outport
  Out1 : Outport  Port=2
  wires:
  In2/1 -> Logical Operator3/1, Logical Operator/1
  In3/1 -> Logical Operator3/2, Logical Operator/2
  Logical Operator/1 -> Logical Operator1/1, Logical Operator2/1
  Logical Operator1/1 -> Out2/1
  Logical Operator4/1 -> Out1/1
  Logical Operator2/1 -> Logical Operator4/1
  Logical Operator3/1 -> Logical Operator4/2
  In4/1 -> Logical Operator2/2, Logical Operator1/2

== system project/ALU2/Subsystem1 ==
  sel2 : Inport
  sel1 : Inport  Port=2
  sel0 : Inport  Port=3
  Add : Sum
  Bit to Integer Converter : commutil2/Bit to Integer Converter  nbits=3  bitOrder=MSB first  signedOutputValues=Unsigned  outDtype=Inherit via internal rule  outDtypeSigned=Inherit via internal rule
  Ground : Ground
  Logical Operator3 : Logic  Operator=NOT  IconShape=distinctive  AllPortsSameDT=off  OutDataTypeStr=boolean
  Mux1 : Mux  Inputs=3
  Out1 : Outport
  wires:
  sel0/1 -> Mux1/3
  Ground/1 -> Logical Operator3/1
  Bit to Integer Converter/1 -> Add/1
  sel1/1 -> Mux1/2
  Mux1/1 -> Bit to Integer Converter/1
  Add/1 -> Out1/1
  Logical Operator3/1 -> Add/2
  sel2/1 -> Mux1/1

== system project/ALU2/cas16 ==
  T : Inport
  rin : Inport  Port=2
  d : Inport  Port=3
  cin : Inport  Port=4
  FA : Subsystem
  Logical Operator : Logic  Operator=XOR  IconShape=distinctive  AllPortsSameDT=off  OutDataTypeStr=boolean
  cout : Outport
  rout : Outport  Port=2
  wires:
  cin/1 -> FA/3(In4)
  rin/1 -> FA/1(In2)
  FA/2(Out1) -> cout/1
  T/1 -> Logical Operator/1
  d/1 -> Logical Operator/2
  Logical Operator/1 -> FA/2(In3)
  FA/1(Out2) -> rout/1

== system project/ALU2/cas17 ==
  T : Inport
  rin : Inport  Port=2
  d : Inport  Port=3
  cin : Inport  Port=4
  FA : Subsystem
  Logical Operator : Logic  Operator=XOR  IconShape=distinctive  AllPortsSameDT=off  OutDataTypeStr=boolean
  cout : Outport
  rout : Outport  Port=2
  wires:
  cin/1 -> FA/3(In4)
  rin/1 -> FA/1(In2)
  FA/2(Out1) -> cout/1
  T/1 -> Logical Operator/1
  d/1 -> Logical Operator/2
  Logical Operator/1 -> FA/2(In3)
  FA/1(Out2) -> rout/1

== system project/ALU2/cas18 ==
  T : Inport
  rin : Inport  Port=2
  d : Inport  Port=3
  cin : Inport  Port=4
  FA : Subsystem
  Logical Operator : Logic  Operator=XOR  IconShape=distinctive  AllPortsSameDT=off  OutDataTypeStr=boolean
  cout : Outport
  rout : Outport  Port=2
  wires:
  cin/1 -> FA/3(In4)
  rin/1 -> FA/1(In2)
  FA/2(Out1) -> cout/1
  T/1 -> Logical Operator/1
  d/1 -> Logical Operator/2
  Logical Operator/1 -> FA/2(In3)
  FA/1(Out2) -> rout/1

== system project/ALU2/cas19 ==
  T : Inport
  rin : Inport  Port=2
  d : Inport  Port=3
  cin : Inport  Port=4
  FA : Subsystem
  Logical Operator : Logic  Operator=XOR  IconShape=distinctive  AllPortsSameDT=off  OutDataTypeStr=boolean
  cout : Outport
  rout : Outport  Port=2
  wires:
  cin/1 -> FA/3(In4)
  rin/1 -> FA/1(In2)
  FA/2(Out1) -> cout/1
  T/1 -> Logical Operator/1
  d/1 -> Logical Operator/2
  Logical Operator/1 -> FA/2(In3)
  FA/1(Out2) -> rout/1

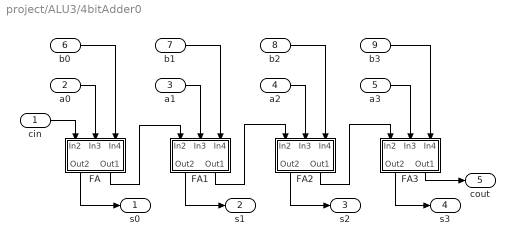
== system project/ALU3/4bitAdder0 ==
  cin : Inport
  a0 : Inport  Port=2
  a1 : Inport  Port=3
  a2 : Inport  Port=4
  a3 : Inport  Port=5
  b0 : Inport  Port=6
  b1 : Inport  Port=7
  b2 : Inport  Port=8
  b3 : Inport  Port=9
  FA : Subsystem
  FA1 : Subsystem
  FA2 : Subsystem
  FA3 : Subsystem
  s0 : Outport
  s1 : Outport  Port=2
  s2 : Outport  Port=3
  s3 : Outport  Port=4
  cout : Outport  Port=5
  wires:
  a2/1 -> FA2/2(In3)
  a0/1 -> FA/2(In3)
  FA2/2(Out1) -> FA3/1(In2)
  b2/1 -> FA2/3(In4)
  b3/1 -> FA3/3(In4)
  cin/1 -> FA/1(In2)
  a3/1 -> FA3/2(In3)
  FA2/1(Out2) -> s2/1
  FA3/1(Out2) -> s3/1
  FA/1(Out2) -> s0/1
  b0/1 -> FA/3(In4)
  a1/1 -> FA1/2(In3)
  FA1/1(Out2) -> s1/1
  FA/2(Out1) -> FA1/1(In2)
  b1/1 -> FA1/3(In4)
  FA1/2(Out1) -> FA2/1(In2)
  FA3/2(Out1) -> cout/1

== system project/ALU3/FA ==
  In2 : Inport
  In3 : Inport  Port=2
  In4 : Inport  Port=3
  Logical Operator : Logic  Operator=XOR  IconShape=distinctive  AllPortsSameDT=off  OutDataTypeStr=boolean
  Logical Operator1 : Logic  Operator=XOR  IconShape=distinctive  AllPortsSameDT=off  OutDataTypeStr=boolean
  Logical Operator2 : Logic  IconShape=distinctive  AllPortsSameDT=off  OutDataTypeStr=boolean
  Logical Operator3 : Logic  IconShape=distinctive  AllPortsSameDT=off  OutDataTypeStr=boolean
  Logical Operator4 : Logic  Operator=OR  IconShape=distinctive  AllPortsSameDT=off  OutDataTypeStr=boolean
  Out2 : Outport
  Out1 : Outport  Port=2
  wires:
  In2/1 -> Logical Operator3/1, Logical Operator/1
  In3/1 -> Logical Operator3/2, Logical Operator/2
  Logical Operator/1 -> Logical Operator1/1, Logical Operator2/1
  Logical Operator1/1 -> Out2/1
  Logical Operator4/1 -> Out1/1
  Logical Operator2/1 -> Logical Operator4/1
  Logical Operator3/1 -> Logical Operator4/2
  In4/1 -> Logical Operator2/2, Logical Operator1/2

== system project/ALU3/Subsystem1 ==
  sel2 : Inport
  sel1 : Inport  Port=2
  sel0 : Inport  Port=3
  Add : Sum
  Bit to Integer Converter : commutil2/Bit to Integer Converter  nbits=3  bitOrder=MSB first  signedOutputValues=Unsigned  outDtype=Inherit via internal rule  outDtypeSigned=Inherit via internal rule
  Ground : Ground
  Logical Operator3 : Logic  Operator=NOT  IconShape=distinctive  AllPortsSameDT=off  OutDataTypeStr=boolean
  Mux1 : Mux  Inputs=3
  Out1 : Outport
  wires:
  sel0/1 -> Mux1/3
  Ground/1 -> Logical Operator3/1
  Bit to Integer Converter/1 -> Add/1
  sel1/1 -> Mux1/2
  Mux1/1 -> Bit to Integer Converter/1
  Add/1 -> Out1/1
  Logical Operator3/1 -> Add/2
  sel2/1 -> Mux1/1

== system project/ALU3/cas16 ==
  T : Inport
  rin : Inport  Port=2
  d : Inport  Port=3
  cin : Inport  Port=4
  FA : Subsystem
  Logical Operator : Logic  Operator=XOR  IconShape=distinctive  AllPortsSameDT=off  OutDataTypeStr=boolean
  cout : Outport
  rout : Outport  Port=2
  wires:
  cin/1 -> FA/3(In4)
  rin/1 -> FA/1(In2)
  FA/2(Out1) -> cout/1
  T/1 -> Logical Operator/1
  d/1 -> Logical Operator/2
  Logical Operator/1 -> FA/2(In3)
  FA/1(Out2) -> rout/1

== system project/ALU3/cas17 ==
  T : Inport
  rin : Inport  Port=2
  d : Inport  Port=3
  cin : Inport  Port=4
  FA : Subsystem
  Logical Operator : Logic  Operator=XOR  IconShape=distinctive  AllPortsSameDT=off  OutDataTypeStr=boolean
  cout : Outport
  rout : Outport  Port=2
  wires:
  cin/1 -> FA/3(In4)
  rin/1 -> FA/1(In2)
  FA/2(Out1) -> cout/1
  T/1 -> Logical Operator/1
  d/1 -> Logical Operator/2
  Logical Operator/1 -> FA/2(In3)
  FA/1(Out2) -> rout/1

== system project/ALU3/cas18 ==
  T : Inport
  rin : Inport  Port=2
  d : Inport  Port=3
  cin : Inport  Port=4
  FA : Subsystem
  Logical Operator : Logic  Operator=XOR  IconShape=distinctive  AllPortsSameDT=off  OutDataTypeStr=boolean
  cout : Outport
  rout : Outport  Port=2
  wires:
  cin/1 -> FA/3(In4)
  rin/1 -> FA/1(In2)
  FA/2(Out1) -> cout/1
  T/1 -> Logical Operator/1
  d/1 -> Logical Operator/2
  Logical Operator/1 -> FA/2(In3)
  FA/1(Out2) -> rout/1

== system project/ALU3/cas19 ==
  T : Inport
  rin : Inport  Port=2
  d : Inport  Port=3
  cin : Inport  Port=4
  FA : Subsystem
  Logical Operator : Logic  Operator=XOR  IconShape=distinctive  AllPortsSameDT=off  OutDataTypeStr=boolean
  cout : Outport
  rout : Outport  Port=2
  wires:
  cin/1 -> FA/3(In4)
  rin/1 -> FA/1(In2)
  FA/2(Out1) -> cout/1
  T/1 -> Logical Operator/1
  d/1 -> Logical Operator/2
  Logical Operator/1 -> FA/2(In3)
  FA/1(Out2) -> rout/1

== system project/ALU0/4bitAdder0/FA ==
  In2 : Inport
  In3 : Inport  Port=2
  In4 : Inport  Port=3
  Logical Operator : Logic  Operator=XOR  IconShape=distinctive  AllPortsSameDT=off  OutDataTypeStr=boolean
  Logical Operator1 : Logic  Operator=XOR  IconShape=distinctive  AllPortsSameDT=off  OutDataTypeStr=boolean
  Logical Operator2 : Logic  IconShape=distinctive  AllPortsSameDT=off  OutDataTypeStr=boolean
  Logical Operator3 : Logic  IconShape=distinctive  AllPortsSameDT=off  OutDataTypeStr=boolean
  Logical Operator4 : Logic  Operator=OR  IconShape=distinctive  AllPortsSameDT=off  OutDataTypeStr=boolean
  Out2 : Outport
  Out1 : Outport  Port=2
  wires:
  Logical Operator2/1 -> Logical Operator4/1
  Logical Operator3/1 -> Logical Operator4/2
  Logical Operator1/1 -> Out2/1
  In4/1 -> Logical Operator2/2, Logical Operator1/2
  In3/1 -> Logical Operator3/2, Logical Operator/2
  In2/1 -> Logical Operator3/1, Logical Operator/1
  Logical Operator/1 -> Logical Operator1/1, Logical Operator2/1
  Logical Operator4/1 -> Out1/1

== system project/ALU0/4bitAdder0/FA1 ==
  In2 : Inport
  In3 : Inport  Port=2
  In4 : Inport  Port=3
  Logical Operator : Logic  Operator=XOR  IconShape=distinctive  AllPortsSameDT=off  OutDataTypeStr=boolean
  Logical Operator1 : Logic  Operator=XOR  IconShape=distinctive  AllPortsSameDT=off  OutDataTypeStr=boolean
  Logical Operator2 : Logic  IconShape=distinctive  AllPortsSameDT=off  OutDataTypeStr=boolean
  Logical Operator3 : Logic  IconShape=distinctive  AllPortsSameDT=off  OutDataTypeStr=boolean
  Logical Operator4 : Logic  Operator=OR  IconShape=distinctive  AllPortsSameDT=off  OutDataTypeStr=boolean
  Out2 : Outport
  Out1 : Outport  Port=2
  wires:
  Logical Operator2/1 -> Logical Operator4/1
  Logical Operator3/1 -> Logical Operator4/2
  Logical Operator1/1 -> Out2/1
  In4/1 -> Logical Operator2/2, Logical Operator1/2
  In3/1 -> Logical Operator3/2, Logical Operator/2
  In2/1 -> Logical Operator3/1, Logical Operator/1
  Logical Operator/1 -> Logical Operator1/1, Logical Operator2/1
  Logical Operator4/1 -> Out1/1

== system project/ALU0/4bitAdder0/FA2 ==
  In2 : Inport
  In3 : Inport  Port=2
  In4 : Inport  Port=3
  Logical Operator : Logic  Operator=XOR  IconShape=distinctive  AllPortsSameDT=off  OutDataTypeStr=boolean
  Logical Operator1 : Logic  Operator=XOR  IconShape=distinctive  AllPortsSameDT=off  OutDataTypeStr=boolean
  Logical Operator2 : Logic  IconShape=distinctive  AllPortsSameDT=off  OutDataTypeStr=boolean
  Logical Operator3 : Logic  IconShape=distinctive  AllPortsSameDT=off  OutDataTypeStr=boolean
  Logical Operator4 : Logic  Operator=OR  IconShape=distinctive  AllPortsSameDT=off  OutDataTypeStr=boolean
  Out2 : Outport
  Out1 : Outport  Port=2
  wires:
  Logical Operator2/1 -> Logical Operator4/1
  Logical Operator3/1 -> Logical Operator4/2
  Logical Operator1/1 -> Out2/1
  In4/1 -> Logical Operator2/2, Logical Operator1/2
  In3/1 -> Logical Operator3/2, Logical Operator/2
  In2/1 -> Logical Operator3/1, Logical Operator/1
  Logical Operator/1 -> Logical Operator1/1, Logical Operator2/1
  Logical Operator4/1 -> Out1/1

== system project/ALU0/4bitAdder0/FA3 ==
  In2 : Inport
  In3 : Inport  Port=2
  In4 : Inport  Port=3
  Logical Operator : Logic  Operator=XOR  IconShape=distinctive  AllPortsSameDT=off  OutDataTypeStr=boolean
  Logical Operator1 : Logic  Operator=XOR  IconShape=distinctive  AllPortsSameDT=off  OutDataTypeStr=boolean
  Logical Operator2 : Logic  IconShape=distinctive  AllPortsSameDT=off  OutDataTypeStr=boolean
  Logical Operator3 : Logic  IconShape=distinctive  AllPortsSameDT=off  OutDataTypeStr=boolean
  Logical Operator4 : Logic  Operator=OR  IconShape=distinctive  AllPortsSameDT=off  OutDataTypeStr=boolean
  Out2 : Outport
  Out1 : Outport  Port=2
  wires:
  Logical Operator2/1 -> Logical Operator4/1
  Logical Operator3/1 -> Logical Operator4/2
  Logical Operator1/1 -> Out2/1
  In4/1 -> Logical Operator2/2, Logical Operator1/2
  In3/1 -> Logical Operator3/2, Logical Operator/2
  In2/1 -> Logical Operator3/1, Logical Operator/1
  Logical Operator/1 -> Logical Operator1/1, Logical Operator2/1
  Logical Operator4/1 -> Out1/1

== system project/ALU0/cas16/FA ==
  In2 : Inport
  In3 : Inport  Port=2
  In4 : Inport  Port=3
  Logical Operator : Logic  Operator=XOR  IconShape=distinctive  AllPortsSameDT=off  OutDataTypeStr=boolean
  Logical Operator1 : Logic  Operator=XOR  IconShape=distinctive  AllPortsSameDT=off  OutDataTypeStr=boolean
  Logical Operator2 : Logic  IconShape=distinctive  AllPortsSameDT=off  OutDataTypeStr=boolean
  Logical Operator3 : Logic  IconShape=distinctive  AllPortsSameDT=off  OutDataTypeStr=boolean
  Logical Operator4 : Logic  Operator=OR  IconShape=distinctive  AllPortsSameDT=off  OutDataTypeStr=boolean
  Out2 : Outport
  Out1 : Outport  Port=2
  wires:
  Logical Operator2/1 -> Logical Operator4/1
  Logical Operator3/1 -> Logical Operator4/2
  Logical Operator1/1 -> Out2/1
  In4/1 -> Logical Operator2/2, Logical Operator1/2
  In3/1 -> Logical Operator3/2, Logical Operator/2
  In2/1 -> Logical Operator3/1, Logical Operator/1
  Logical Operator/1 -> Logical Operator1/1, Logical Operator2/1
  Logical Operator4/1 -> Out1/1

== system project/ALU0/cas17/FA ==
  In2 : Inport
  In3 : Inport  Port=2
  In4 : Inport  Port=3
  Logical Operator : Logic  Operator=XOR  IconShape=distinctive  AllPortsSameDT=off  OutDataTypeStr=boolean
  Logical Operator1 : Logic  Operator=XOR  IconShape=distinctive  AllPortsSameDT=off  OutDataTypeStr=boolean
  Logical Operator2 : Logic  IconShape=distinctive  AllPortsSameDT=off  OutDataTypeStr=boolean
  Logical Operator3 : Logic  IconShape=distinctive  AllPortsSameDT=off  OutDataTypeStr=boolean
  Logical Operator4 : Logic  Operator=OR  IconShape=distinctive  AllPortsSameDT=off  OutDataTypeStr=boolean
  Out2 : Outport
  Out1 : Outport  Port=2
  wires:
  Logical Operator2/1 -> Logical Operator4/1
  Logical Operator3/1 -> Logical Operator4/2
  Logical Operator1/1 -> Out2/1
  In4/1 -> Logical Operator2/2, Logical Operator1/2
  In3/1 -> Logical Operator3/2, Logical Operator/2
  In2/1 -> Logical Operator3/1, Logical Operator/1
  Logical Operator/1 -> Logical Operator1/1, Logical Operator2/1
  Logical Operator4/1 -> Out1/1

== system project/ALU0/cas18/FA ==
  In2 : Inport
  In3 : Inport  Port=2
  In4 : Inport  Port=3
  Logical Operator : Logic  Operator=XOR  IconShape=distinctive  AllPortsSameDT=off  OutDataTypeStr=boolean
  Logical Operator1 : Logic  Operator=XOR  IconShape=distinctive  AllPortsSameDT=off  OutDataTypeStr=boolean
  Logical Operator2 : Logic  IconShape=distinctive  AllPortsSameDT=off  OutDataTypeStr=boolean
  Logical Operator3 : Logic  IconShape=distinctive  AllPortsSameDT=off  OutDataTypeStr=boolean
  Logical Operator4 : Logic  Operator=OR  IconShape=distinctive  AllPortsSameDT=off  OutDataTypeStr=boolean
  Out2 : Outport
  Out1 : Outport  Port=2
  wires:
  Logical Operator2/1 -> Logical Operator4/1
  Logical Operator3/1 -> Logical Operator4/2
  Logical Operator1/1 -> Out2/1
  In4/1 -> Logical Operator2/2, Logical Operator1/2
  In3/1 -> Logical Operator3/2, Logical Operator/2
  In2/1 -> Logical Operator3/1, Logical Operator/1
  Logical Operator/1 -> Logical Operator1/1, Logical Operator2/1
  Logical Operator4/1 -> Out1/1

== system project/ALU0/cas19/FA ==
  In2 : Inport
  In3 : Inport  Port=2
  In4 : Inport  Port=3
  Logical Operator : Logic  Operator=XOR  IconShape=distinctive  AllPortsSameDT=off  OutDataTypeStr=boolean
  Logical Operator1 : Logic  Operator=XOR  IconShape=distinctive  AllPortsSameDT=off  OutDataTypeStr=boolean
  Logical Operator2 : Logic  IconShape=distinctive  AllPortsSameDT=off  OutDataTypeStr=boolean
  Logical Operator3 : Logic  IconShape=distinctive  AllPortsSameDT=off  OutDataTypeStr=boolean
  Logical Operator4 : Logic  Operator=OR  IconShape=distinctive  AllPortsSameDT=off  OutDataTypeStr=boolean
  Out2 : Outport
  Out1 : Outport  Port=2
  wires:
  Logical Operator2/1 -> Logical Operator4/1
  Logical Operator3/1 -> Logical Operator4/2
  Logical Operator1/1 -> Out2/1
  In4/1 -> Logical Operator2/2, Logical Operator1/2
  In3/1 -> Logical Operator3/2, Logical Operator/2
  In2/1 -> Logical Operator3/1, Logical Operator/1
  Logical Operator/1 -> Logical Operator1/1, Logical Operator2/1
  Logical Operator4/1 -> Out1/1

== system project/ALU1/4bitAdder0/FA ==
  In2 : Inport
  In3 : Inport  Port=2
  In4 : Inport  Port=3
  Logical Operator : Logic  Operator=XOR  IconShape=distinctive  AllPortsSameDT=off  OutDataTypeStr=boolean
  Logical Operator1 : Logic  Operator=XOR  IconShape=distinctive  AllPortsSameDT=off  OutDataTypeStr=boolean
  Logical Operator2 : Logic  IconShape=distinctive  AllPortsSameDT=off  OutDataTypeStr=boolean
  Logical Operator3 : Logic  IconShape=distinctive  AllPortsSameDT=off  OutDataTypeStr=boolean
  Logical Operator4 : Logic  Operator=OR  IconShape=distinctive  AllPortsSameDT=off  OutDataTypeStr=boolean
  Out2 : Outport
  Out1 : Outport  Port=2
  wires:
  Logical Operator2/1 -> Logical Operator4/1
  Logical Operator3/1 -> Logical Operator4/2
  Logical Operator1/1 -> Out2/1
  In4/1 -> Logical Operator2/2, Logical Operator1/2
  In3/1 -> Logical Operator3/2, Logical Operator/2
  In2/1 -> Logical Operator3/1, Logical Operator/1
  Logical Operator/1 -> Logical Operator1/1, Logical Operator2/1
  Logical Operator4/1 -> Out1/1

== system project/ALU1/4bitAdder0/FA1 ==
  In2 : Inport
  In3 : Inport  Port=2
  In4 : Inport  Port=3
  Logical Operator : Logic  Operator=XOR  IconShape=distinctive  AllPortsSameDT=off  OutDataTypeStr=boolean
  Logical Operator1 : Logic  Operator=XOR  IconShape=distinctive  AllPortsSameDT=off  OutDataTypeStr=boolean
  Logical Operator2 : Logic  IconShape=distinctive  AllPortsSameDT=off  OutDataTypeStr=boolean
  Logical Operator3 : Logic  IconShape=distinctive  AllPortsSameDT=off  OutDataTypeStr=boolean
  Logical Operator4 : Logic  Operator=OR  IconShape=distinctive  AllPortsSameDT=off  OutDataTypeStr=boolean
  Out2 : Outport
  Out1 : Outport  Port=2
  wires:
  Logical Operator2/1 -> Logical Operator4/1
  Logical Operator3/1 -> Logical Operator4/2
  Logical Operator1/1 -> Out2/1
  In4/1 -> Logical Operator2/2, Logical Operator1/2
  In3/1 -> Logical Operator3/2, Logical Operator/2
  In2/1 -> Logical Operator3/1, Logical Operator/1
  Logical Operator/1 -> Logical Operator1/1, Logical Operator2/1
  Logical Operator4/1 -> Out1/1

== system project/ALU1/4bitAdder0/FA2 ==
  In2 : Inport
  In3 : Inport  Port=2
  In4 : Inport  Port=3
  Logical Operator : Logic  Operator=XOR  IconShape=distinctive  AllPortsSameDT=off  OutDataTypeStr=boolean
  Logical Operator1 : Logic  Operator=XOR  IconShape=distinctive  AllPortsSameDT=off  OutDataTypeStr=boolean
  Logical Operator2 : Logic  IconShape=distinctive  AllPortsSameDT=off  OutDataTypeStr=boolean
  Logical Operator3 : Logic  IconShape=distinctive  AllPortsSameDT=off  OutDataTypeStr=boolean
  Logical Operator4 : Logic  Operator=OR  IconShape=distinctive  AllPortsSameDT=off  OutDataTypeStr=boolean
  Out2 : Outport
  Out1 : Outport  Port=2
  wires:
  Logical Operator2/1 -> Logical Operator4/1
  Logical Operator3/1 -> Logical Operator4/2
  Logical Operator1/1 -> Out2/1
  In4/1 -> Logical Operator2/2, Logical Operator1/2
  In3/1 -> Logical Operator3/2, Logical Operator/2
  In2/1 -> Logical Operator3/1, Logical Operator/1
  Logical Operator/1 -> Logical Operator1/1, Logical Operator2/1
  Logical Operator4/1 -> Out1/1

== system project/ALU1/4bitAdder0/FA3 ==
  In2 : Inport
  In3 : Inport  Port=2
  In4 : Inport  Port=3
  Logical Operator : Logic  Operator=XOR  IconShape=distinctive  AllPortsSameDT=off  OutDataTypeStr=boolean
  Logical Operator1 : Logic  Operator=XOR  IconShape=distinctive  AllPortsSameDT=off  OutDataTypeStr=boolean
  Logical Operator2 : Logic  IconShape=distinctive  AllPortsSameDT=off  OutDataTypeStr=boolean
  Logical Operator3 : Logic  IconShape=distinctive  AllPortsSameDT=off  OutDataTypeStr=boolean
  Logical Operator4 : Logic  Operator=OR  IconShape=distinctive  AllPortsSameDT=off  OutDataTypeStr=boolean
  Out2 : Outport
  Out1 : Outport  Port=2
  wires:
  Logical Operator2/1 -> Logical Operator4/1
  Logical Operator3/1 -> Logical Operator4/2
  Logical Operator1/1 -> Out2/1
  In4/1 -> Logical Operator2/2, Logical Operator1/2
  In3/1 -> Logical Operator3/2, Logical Operator/2
  In2/1 -> Logical Operator3/1, Logical Operator/1
  Logical Operator/1 -> Logical Operator1/1, Logical Operator2/1
  Logical Operator4/1 -> Out1/1

== system project/ALU1/cas16/FA ==
  In2 : Inport
  In3 : Inport  Port=2
  In4 : Inport  Port=3
  Logical Operator : Logic  Operator=XOR  IconShape=distinctive  AllPortsSameDT=off  OutDataTypeStr=boolean
  Logical Operator1 : Logic  Operator=XOR  IconShape=distinctive  AllPortsSameDT=off  OutDataTypeStr=boolean
  Logical Operator2 : Logic  IconShape=distinctive  AllPortsSameDT=off  OutDataTypeStr=boolean
  Logical Operator3 : Logic  IconShape=distinctive  AllPortsSameDT=off  OutDataTypeStr=boolean
  Logical Operator4 : Logic  Operator=OR  IconShape=distinctive  AllPortsSameDT=off  OutDataTypeStr=boolean
  Out2 : Outport
  Out1 : Outport  Port=2
  wires:
  Logical Operator2/1 -> Logical Operator4/1
  Logical Operator3/1 -> Logical Operator4/2
  Logical Operator1/1 -> Out2/1
  In4/1 -> Logical Operator2/2, Logical Operator1/2
  In3/1 -> Logical Operator3/2, Logical Operator/2
  In2/1 -> Logical Operator3/1, Logical Operator/1
  Logical Operator/1 -> Logical Operator1/1, Logical Operator2/1
  Logical Operator4/1 -> Out1/1

== system project/ALU1/cas17/FA ==
  In2 : Inport
  In3 : Inport  Port=2
  In4 : Inport  Port=3
  Logical Operator : Logic  Operator=XOR  IconShape=distinctive  AllPortsSameDT=off  OutDataTypeStr=boolean
  Logical Operator1 : Logic  Operator=XOR  IconShape=distinctive  AllPortsSameDT=off  OutDataTypeStr=boolean
  Logical Operator2 : Logic  IconShape=distinctive  AllPortsSameDT=off  OutDataTypeStr=boolean
  Logical Operator3 : Logic  IconShape=distinctive  AllPortsSameDT=off  OutDataTypeStr=boolean
  Logical Operator4 : Logic  Operator=OR  IconShape=distinctive  AllPortsSameDT=off  OutDataTypeStr=boolean
  Out2 : Outport
  Out1 : Outport  Port=2
  wires:
  Logical Operator2/1 -> Logical Operator4/1
  Logical Operator3/1 -> Logical Operator4/2
  Logical Operator1/1 -> Out2/1
  In4/1 -> Logical Operator2/2, Logical Operator1/2
  In3/1 -> Logical Operator3/2, Logical Operator/2
  In2/1 -> Logical Operator3/1, Logical Operator/1
  Logical Operator/1 -> Logical Operator1/1, Logical Operator2/1
  Logical Operator4/1 -> Out1/1
